simulink library "csu_trh_tracker_head_lib"  (R2014b)
settings: Solver=ode45  SolverMode=SingleTasking  StartTime=0.0  StopTime=10.0  RelTol=1e-3
values from neighbouring files (symbols this model uses):
  sim_time_step_size = 0.01    [csu_lak_linear_accel_kinematics_test.m]
undefined symbols (not defined in the file or in its folder): sta_rate_max
libraries: util_common_lib x7, util_quat_lib x3, simulink x1, util_info_lib x1
settings Model: Creator=eleanor  LastModifiedBy=mstewart

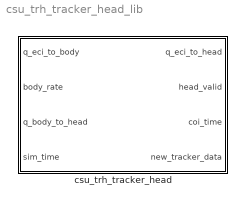
== system csu_trh_tracker_head_lib ==
  csu_trh_tracker_head : Subsystem  SystemSampleTime=0.1
  wires:
  ? -> csu_trh_tracker_head/1(q_eci_to_body)  "rrk_q_body_from_eci"

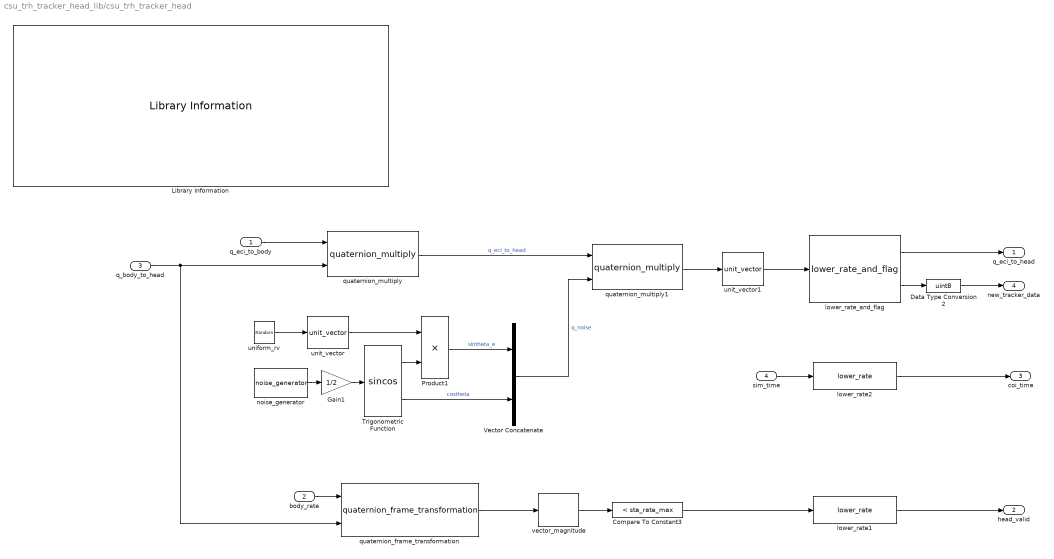
== system csu_trh_tracker_head_lib/csu_trh_tracker_head ==
  q_eci_to_body : Inport
  body_rate : Inport  Port=2
  q_body_to_head : Inport  Port=3
  sim_time : Inport  Port=4
  Compare To Constant3 : simulink/Logic and Bit Operations/Compare To Constant  relop=<  const=sta_rate_max  OutDataTypeStr=uint8
  Data Type Conversion2 : DataTypeConversion  OutDataTypeStr=uint8
  Gain1 : Gain  Gain=1/2
  Library Information : util_info_lib/Library Information  owner='NONE'
  Product1 : Product  RndMeth=Zero
  Trigonometric Function : Trigonometry  Operator=sincos
  Vector Concatenate : Concatenate
  lower_rate1 : util_common_lib/lower_rate  counter_max=sta_att_counter  counter_init=0
  lower_rate2 : util_common_lib/lower_rate  counter_max=sta_att_counter  counter_init=0
  lower_rate_and_flag : util_common_lib/lower_rate_and_flag  counter_max=sta_att_counter  counter_init=0
  noise_generator : util_common_lib/noise_generator  std_dev=sta_angle_std  bias=sta_angle_bias  seed=sta_angle_seed  on=1  sample_time=sim_time_step_size
  quaternion_frame_transformation : util_quat_lib/quaternion_frame_transformation  SystemSampleTime=-1
  quaternion_multiply : util_quat_lib/quaternion_multiply  SystemSampleTime=-1
  quaternion_multiply1 : util_quat_lib/quaternion_multiply  SystemSampleTime=-1
  uniform_rv : UniformRandomNumber  Minimum=[-1 -1 -1]  Maximum=[1 1 1]  SampleTime=sim_time_step_size
  unit_vector : util_common_lib/unit_vector  SystemSampleTime=-1
  unit_vector1 : util_common_lib/unit_vector  SystemSampleTime=-1
  vector_magnitude : util_common_lib/vector_magnitude  SystemSampleTime=-1
  q_eci_to_head : Outport
  head_valid : Outport  Port=2
  coi_time : Outport  Port=3
  new_tracker_data : Outport  Port=4
  wires:
  Compare To Constant3/1 -> lower_rate1/1
  vector_magnitude/1 -> Compare To Constant3/1
  quaternion_frame_transformation/1 -> vector_magnitude/1
  body_rate/1 -> quaternion_frame_transformation/1
  quaternion_multiply1/1 -> unit_vector1/1
  Vector Concatenate/1 -> quaternion_multiply1/2  "q_noise"
  Gain1/1 -> Trigonometric Function/1
  Product1/1 -> Vector Concatenate/1  "sintheta_e"
  unit_vector/1 -> Product1/1
  Trigonometric Function/2 -> Vector Concatenate/2  "costheta"
  Trigonometric Function/1 -> Product1/2
  noise_generator/1 -> Gain1/1
  uniform_rv/1 -> unit_vector/1
  quaternion_multiply/1 -> quaternion_multiply1/1  "q_eci_to_head"
  q_body_to_head/1 -> quaternion_multiply/2, quaternion_frame_transformation/2
  q_eci_to_body/1 -> quaternion_multiply/1
  lower_rate_and_flag/2 -> Data Type Conversion2/1
  lower_rate_and_flag/1 -> q_eci_to_head/1
  unit_vector1/1 -> lower_rate_and_flag/1
  lower_rate1/1 -> head_valid/1
  Data Type Conversion2/1 -> new_tracker_data/1
  sim_time/1 -> lower_rate2/1
  lower_rate2/1 -> coi_time/1
